simulink model "main2"  (R2024a)
settings: Solver=ode15s  StartTime=0.0  StopTime=2  MaxStep=1e-4  RelTol=1e-3
InitFcn:
  | parametros
values from neighbouring files (symbols this model uses):
  alpha_cu = 3.9 *10^-3    (= 0.0039)    [parametros.m]
  b_l = 0.1    [parametros.m]
  b_m = 1.5 * 10^-5    (= 1.5e-05)    [parametros.m]
  C_ts = 0.818    [parametros.m]
  J_l = (m*l_cm^2 + J_cm) + (m_l * l_l^2)    (= 0.0833)    [parametros.m]
  J_m = 1.4 * 10^-5    (= 1.4e-05)    [parametros.m]
  k_l = m * g * l_cm + m_l * g * l_l    (= 2.4516625)    [parametros.m]
  L_d = 6.6 * 10^-3    (= 0.0066)    [parametros.m]
  L_ls = 0.8 * 10^-3    (= 0.0008)    [parametros.m]
  L_q = 5.8 * 10^-3    (= 0.0058)    [parametros.m]
  lambda_m = 0.016    [parametros.m]
  P_p = 3    [parametros.m]
  r = 120    [parametros.m]
  R_s_40 = 1.02    [parametros.m]
  R_ts_amb = 146.7    [parametros.m]
  Temp_s_ref = 40    [parametros.m]
undefined symbols (not defined in the file or in its folder): K_e_omega, K_e_theta
libraries: simulink x6
(part 2 of 2)

== matlab function main2/5.2.1 ids = 0/TD_PARK ==
  data: fas input; fqs output; fbs input; fcs input; theta_r input; fds output; f0s output
function [fqs, fds, f0s] = TD_PARK(fas, fbs, fcs, theta_r)

    fabcs = [fas; fbs; fcs];

    Ks = 2/3*[cos(theta_r) cos(theta_r - 2*pi/3) cos(theta_r + 2*pi/3)
          sin(theta_r) sin(theta_r - 2*pi/3) sin(theta_r + 2*pi/3) 
          1/2          1/2                   1/2];

    fqd0s = Ks * fabcs;

    fqs = fqd0s(1);
    fds = fqd0s(2);
    f0s = fqd0s(3);

end

== matlab function main2/5.2.1 ids = 1/TD_PARK ==
  data: fas input; fqs output; fbs input; fcs input; theta_r input; fds output; f0s output
function [fqs, fds, f0s] = TD_PARK(fas, fbs, fcs, theta_r)

    fabcs = [fas; fbs; fcs];

    Ks = 2/3*[cos(theta_r) cos(theta_r - 2*pi/3) cos(theta_r + 2*pi/3)
          sin(theta_r) sin(theta_r - 2*pi/3) sin(theta_r + 2*pi/3) 
          1/2          1/2                   1/2];

    fqd0s = Ks * fabcs;

    fqs = fqd0s(1);
    fds = fqd0s(2);
    f0s = fqd0s(3);

end

== matlab function main2/5.2.1 ids = 1/TI_PARK1 ==
  data: fqs input; fas output; fds input; f0s input; theta_r input; fbs output; fcs output
function [fas, fbs, fcs] = TI_PARK(fqs, fds, f0s , theta_r)

    fqd0s = [fqs; fds; f0s];

    Ks = [cos(theta_r)         sin(theta_r)             1
          cos(theta_r - 2*pi/3) sin(theta_r - 2*pi/3)    1
          cos(theta_r + 2*pi/3) sin(theta_r + 2*pi/3)    1];

    fabcs = Ks * fqd0s;

    fas = fabcs(1);
    fbs = fabcs(2);
    fcs = fabcs(3);

end

== matlab function main2/5.2.1 ids = 0/Subsistema físico no lineal /TI_PARK ==
  data: fqs input; fas output; fds input; f0s input; theta_r input; fbs output; fcs output
function [fas, fbs, fcs] = TI_PARK(fqs, fds, f0s , theta_r)

    fqd0s = [fqs; fds; f0s];

    Ks = [cos(theta_r)         sin(theta_r)             1
          cos(theta_r - 2*pi/3) sin(theta_r - 2*pi/3)    1
          cos(theta_r + 2*pi/3) sin(theta_r + 2*pi/3)    1];

    fabcs = Ks * fqd0s;

    fas = fabcs(1);
    fbs = fabcs(2);
    fcs = fabcs(3);

end

== matlab function main2/5.2.1 ids = 2/Subsistema físico no lineal /TD_PARK ==
  data: fas input; fqs output; fbs input; fcs input; theta_r input; fds output; f0s output
function [fqs, fds, f0s] = TD_PARK(fas, fbs, fcs, theta_r)

    fabcs = [fas; fbs; fcs];

    Ks = 2/3*[cos(theta_r) cos(theta_r - 2*pi/3) cos(theta_r + 2*pi/3)
          sin(theta_r) sin(theta_r - 2*pi/3) sin(theta_r + 2*pi/3) 
          1/2          1/2                   1/2];

    fqd0s = Ks * fabcs;

    fqs = fqd0s(1);
    fds = fqd0s(2);
    f0s = fqd0s(3);

end

== matlab function main2/5.2.1 ids = 2/Subsistema físico no lineal /TI_PARK ==
  data: fqs input; fas output; fds input; f0s input; theta_r input; fbs output; fcs output
function [fas, fbs, fcs] = TI_PARK(fqs, fds, f0s , theta_r)

    fqd0s = [fqs; fds; f0s];

    Ks = [cos(theta_r)         sin(theta_r)             1
          cos(theta_r - 2*pi/3) sin(theta_r - 2*pi/3)    1
          cos(theta_r + 2*pi/3) sin(theta_r + 2*pi/3)    1];

    fabcs = Ks * fqd0s;

    fas = fabcs(1);
    fbs = fabcs(2);
    fcs = fabcs(3);

end

== matlab function main2/5.2.1 ids = 2/TD_PARK ==
  data: fas input; fqs output; fbs input; fcs input; theta_r input; fds output; f0s output
function [fqs, fds, f0s] = TD_PARK(fas, fbs, fcs, theta_r)

    fabcs = [fas; fbs; fcs];

    Ks = 2/3*[cos(theta_r) cos(theta_r - 2*pi/3) cos(theta_r + 2*pi/3)
          sin(theta_r) sin(theta_r - 2*pi/3) sin(theta_r + 2*pi/3) 
          1/2          1/2                   1/2];

    fqd0s = Ks * fabcs;

    fqs = fqd0s(1);
    fds = fqd0s(2);
    f0s = fqd0s(3);

end

== matlab function main2/5.2.1 ids = 2/TI_PARK1 ==
  data: fqs input; fas output; fds input; f0s input; theta_r input; fbs output; fcs output
function [fas, fbs, fcs] = TI_PARK(fqs, fds, f0s , theta_r)

    fqd0s = [fqs; fds; f0s];

    Ks = [cos(theta_r)         sin(theta_r)             1
          cos(theta_r - 2*pi/3) sin(theta_r - 2*pi/3)    1
          cos(theta_r + 2*pi/3) sin(theta_r + 2*pi/3)    1];

    fabcs = Ks * fqd0s;

    fas = fabcs(1);
    fbs = fabcs(2);
    fcs = fabcs(3);

end

== matlab function main2/5.2.1 ids = 1/Subsistema físico no lineal /TD_PARK ==
  data: fas input; fqs output; fbs input; fcs input; theta_r input; fds output; f0s output
function [fqs, fds, f0s] = TD_PARK(fas, fbs, fcs, theta_r)

    fabcs = [fas; fbs; fcs];

    Ks = 2/3*[cos(theta_r) cos(theta_r - 2*pi/3) cos(theta_r + 2*pi/3)
          sin(theta_r) sin(theta_r - 2*pi/3) sin(theta_r + 2*pi/3) 
          1/2          1/2                   1/2];

    fqd0s = Ks * fabcs;

    fqs = fqd0s(1);
    fds = fqd0s(2);
    f0s = fqd0s(3);

end

== matlab function main2/5.2.1 ids = 1/Subsistema físico no lineal /TI_PARK ==
  data: fqs input; fas output; fds input; f0s input; theta_r input; fbs output; fcs output
function [fas, fbs, fcs] = TI_PARK(fqs, fds, f0s , theta_r)

    fqd0s = [fqs; fds; f0s];

    Ks = [cos(theta_r)         sin(theta_r)             1
          cos(theta_r - 2*pi/3) sin(theta_r - 2*pi/3)    1
          cos(theta_r + 2*pi/3) sin(theta_r + 2*pi/3)    1];

    fabcs = Ks * fqd0s;

    fas = fabcs(1);
    fbs = fabcs(2);
    fcs = fabcs(3);

end
